simulink model "dpcm"  (R2018b)
settings: Solver=VariableStepAuto  StartTime=0.0  StopTime=10.0  RelTol=1e-3
libraries: dspquant2 x2, dsparch4 x1, commutil2 x1
settings Model: Creator=shahb  LastModifiedBy=shahb
settings DebuggingCC: LibraryContextMissingDiagnostic=none
settings SFSimCC: SimUseLocalCustomCode=off
settings RTWCC: RTWUseLocalCustomCode=off

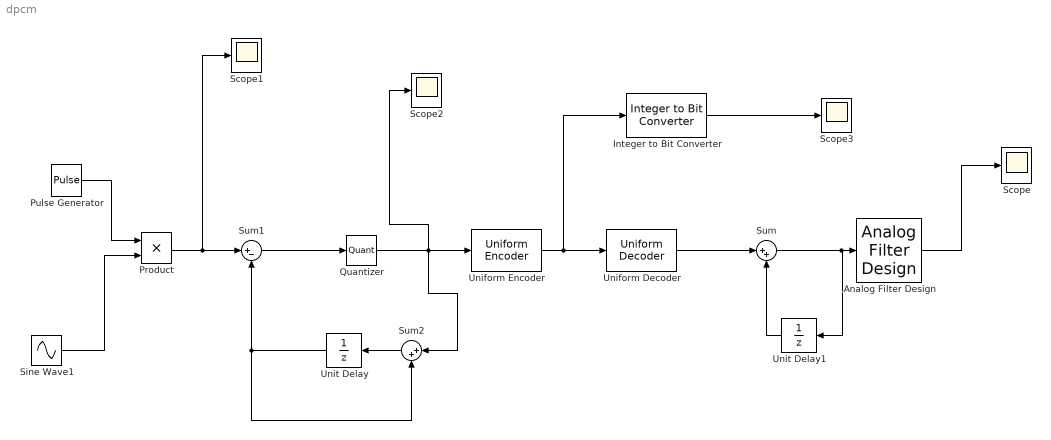
== system dpcm ==
  Analog Filter Design : dsparch4/Analog Filter Design  method=Bessel  filttype=Lowpass  N=8  Wlo=10*pi  Whi=80  Rp=2  Rs=40
  Integer to Bit Converter : commutil2/Integer to Bit Converter  nbits=12  signedInputValues=Signed  bitOrder=MSB first  outDtype=Inherit via internal rule
  Product : Product
  Pulse Generator : DiscretePulseGenerator  PulseType=Time based  Period=0.05  PulseWidth=50
  Quantizer : Quantizer  QuantizationInterval=0.005
  Scope{,1..3} (4 alike) : Scope
  Sine Wave1 : Sin  Frequency=2  SampleTime=0
  Sum : Sum  Inputs=|++
  Sum1 : Sum  Inputs=|+-
  Sum2 : Sum  Inputs=|++
  Uniform Decoder : dspquant2/Uniform Decoder  peak=1  bits=12  overflowMode=Saturate  otype=Double
      settings: SourceProductName=DSP System Toolbox  SourceProductBaseCode=DS
  Uniform Encoder : dspquant2/Uniform Encoder  peak=1  bits=12  otype=Signed integer
      settings: SourceProductName=DSP System Toolbox
  Unit Delay : UnitDelay  SampleTime=-1
  Unit Delay1 : UnitDelay  SampleTime=-1
  wires:
  Sine Wave1/1 -> Product/2
  Pulse Generator/1 -> Product/1
  Product/1 -> Scope1/1, Sum1/1
  Quantizer/1 -> Scope2/1, Uniform Encoder/1, Sum2/1
  Uniform Decoder/1 -> Sum/1
  Sum/1 -> Unit Delay1/1, Analog Filter Design/1
  Sum2/1 -> Unit Delay/1
  Unit Delay/1 -> Sum1/2, Sum2/2
  Unit Delay1/1 -> Sum/2
  Uniform Encoder/1 -> Integer to Bit Converter/1, Uniform Decoder/1
  Sum1/1 -> Quantizer/1
  Analog Filter Design/1 -> Scope/1
  Integer to Bit Converter/1 -> Scope3/1
